simulink model "Q_Car_RL_TD3_Road_Signal"  (R2020b)
settings: Solver=VariableStepAuto  StartTime=0.0  StopTime=4  RelTol=1e-3
values from neighbouring files (symbols this model uses):
  b1 = 2126    [ModelParameters.mat]
  b2 = 1000    [ModelParameters.mat]
  Gqn0 = 4096 X 10^-6 (0.004096)    [RoadParameters.m]
  k1 = 24000    [ModelParameters.mat]
  k2 = 350000    [ModelParameters.mat]
  m1 = 365    [ModelParameters.mat]
  m2 = 43    [ModelParameters.mat]
  P_Noise = 28.5    [RoadParameters.m]
  Ts = 0.001    [Agent_Run.m]    (also in Learning_Algorithm_TD3.m)
undefined symbols (not defined in the file or in its folder): DiscIntNeverNeededParam, magnitude
libraries: simulink x4, rllib x1
settings Model: Creator=Administrator  LastModifiedBy=cloud
settings SolverCC: ZeroCrossAlgorithm=Adaptive
settings DebuggingCC: MaskedZcDiagnostic=none  IgnoredZcDiagnostic=none

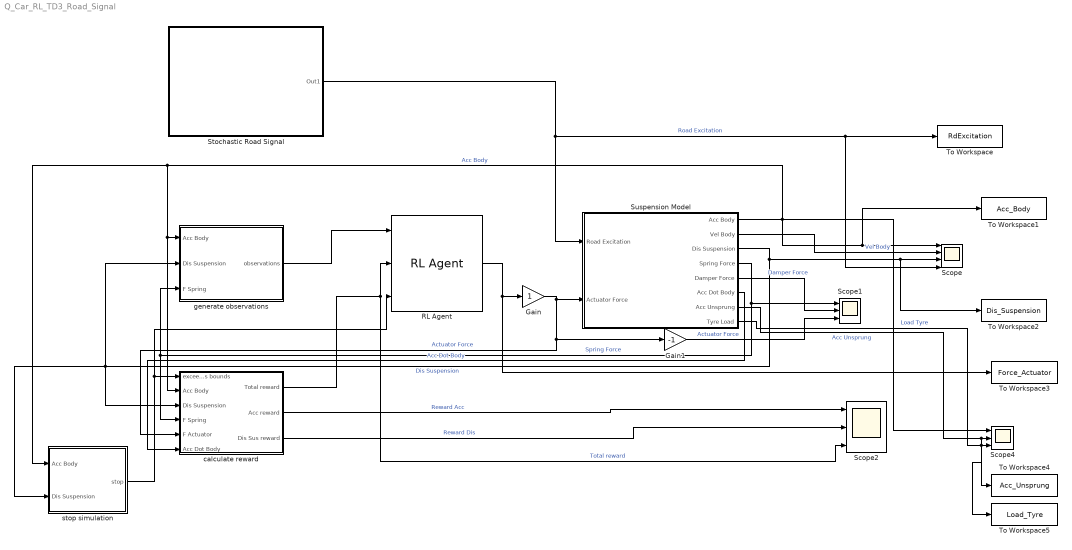
== system Q_Car_RL_TD3_Road_Signal ==
  Gain : Gain
  Gain1 : Gain  Gain=-1
  RL Agent : rllib/RL Agent  Agent=agent  ProvideReward=on  ProvideIsDone=on  ProvideCumRwd=off  TreatAsDirectFeedthrough=on  CollectLoggedSignals=on  CollectModelStates=on
  Scope : Scope  NumInputPorts=4
  Scope1 : Scope  NumInputPorts=3
  Scope2 : Scope  NumInputPorts=3
  Scope4 : Scope  NumInputPorts=3
  Stochastic Road Signal : Subsystem
  Suspension Model : Subsystem
  To Workspace : ToWorkspace  VariableName=RdExcitation  SaveFormat=Timeseries  SampleTime=0.001
  To Workspace1 : ToWorkspace  VariableName=Acc_Body  SaveFormat=Timeseries  SampleTime=0.001
  To Workspace2 : ToWorkspace  VariableName=Dis_Suspension  SaveFormat=Timeseries  SampleTime=0.001
  To Workspace3 : ToWorkspace  VariableName=Force_Actuator  SaveFormat=Structure With Time  SampleTime=0.001
  To Workspace4 : ToWorkspace  VariableName=Acc_Unsprung  SaveFormat=Timeseries  SampleTime=0.001
  To Workspace5 : ToWorkspace  VariableName=Load_Tyre  SaveFormat=Structure With Time  SampleTime=0.001
  calculate reward : Subsystem
  generate observations : Subsystem
  stop simulation : Subsystem
  wires:
  Suspension Model/1(Acc Body) -> Scope/1, To Workspace1/1, calculate reward/2(Acc Body), generate observations/1(Acc Body), stop simulation/1(Acc Body), Scope4/1  "Acc Body"
  Suspension Model/3(Dis Suspension) -> Scope/3, To Workspace2/1, calculate reward/3(Dis Suspension), stop simulation/2(Dis Suspension), generate observations/2(Dis Suspension)  "Dis Suspension"
  Stochastic Road Signal/1(Out1) -> To Workspace/1, Scope/4, Suspension Model/1(Road Excitation)  "Road Excitation"
  generate observations/1(observations) -> RL Agent/1
  calculate reward/1(Total reward) -> Scope2/3, RL Agent/2  "Total reward"
  stop simulation/1(stop) -> calculate reward/1(exceeds bounds), RL Agent/3
  RL Agent/1 -> Gain/1, To Workspace3/1
  Gain/1 -> Gain1/1, calculate reward/5(F Actuator), Suspension Model/2(Actuator Force)  "Actuator Force"
  Suspension Model/4(Spring Force) -> calculate reward/4(F Spring), generate observations/3(F Spring), Scope1/1  "Spring Force"
  Suspension Model/5(Damper Force) -> Scope1/2  "Damper Force"
  Suspension Model/6(Acc Dot Body) -> calculate reward/6(Acc Dot Body)  "Acc Dot Body"
  calculate reward/2(Acc reward) -> Scope2/1  "Reward Acc"
  calculate reward/3(Dis Sus reward) -> Scope2/2  "Reward Dis"
  Gain1/1 -> Scope1/3  "Actuator Force"
  Suspension Model/2(Vel Body) -> Scope/2  "Vel Body"
  Suspension Model/7(Acc Unsprung) -> To Workspace4/1, Scope4/2  "Acc Unsprung"
  Suspension Model/8(Tyre Load) -> To Workspace5/1, Scope4/3  "Load Tyre"

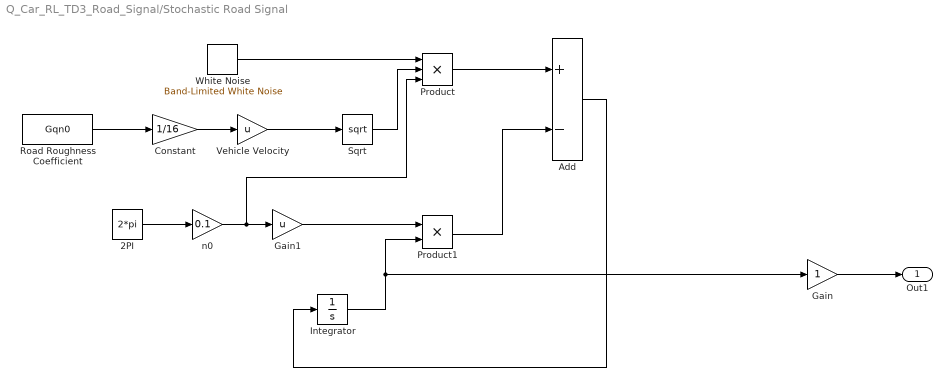
== system Q_Car_RL_TD3_Road_Signal/Stochastic Road Signal ==
  2PI : Constant  Value=2*pi
  Add : Sum  Inputs=+-
  Constant : Gain  Gain=1/16
  Gain : Gain
  Gain1 : Gain  Gain=u
  Integrator : Integrator
  Product : Product  Inputs=3
  Product1 : Product
  Road Roughness Coefficient : Constant  Value=Gqn0
  Sqrt : Sqrt  SaturateOnIntegerOverflow=on
  Vehicle Velocity : Gain  Gain=u
  White Noise : simulink/Sources/Band-Limited White Noise  Cov=[P_Noise]  Ts=0.001  seed=[23341]
  n0 : Gain  Gain=0.1
  Out1 : Outport
  wires:
  Integrator/1 -> Product1/2, Gain/1
  White Noise/1 -> Product/1
  2PI/1 -> n0/1
  n0/1 -> Product/3, Gain1/1
  Gain1/1 -> Product1/1
  Road Roughness Coefficient/1 -> Constant/1
  Gain/1 -> Out1/1
  Constant/1 -> Vehicle Velocity/1
  Add/1 -> Integrator/1
  Product/1 -> Add/1
  Product1/1 -> Add/2
  Sqrt/1 -> Product/2
  Vehicle Velocity/1 -> Sqrt/1

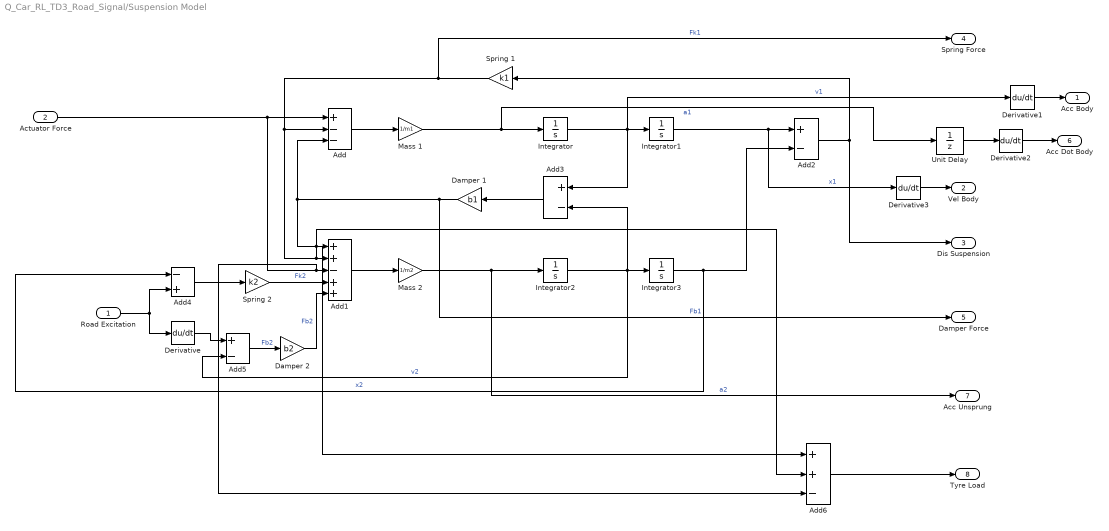
== system Q_Car_RL_TD3_Road_Signal/Suspension Model ==
  Road Excitation : Inport
  Actuator Force : Inport  Port=2
  Add : Sum  Inputs=+--
  Add1 : Sum  Inputs=++-++
  Add2 : Sum  Inputs=+-
  Add3 : Sum  Inputs=+-
  Add4 : Sum  Inputs=-+
  Add5 : Sum  Inputs=+-
  Add6 : Sum  Inputs=++-
  Damper 1 : Gain  Gain=b1
  Damper 2 : Gain  Gain=b2
  Derivative{,1..3} (4 alike) : Derivative
  Integrator{,1..3} (4 alike) : Integrator
  Mass 1 : Gain  Gain=1/m1
  Mass 2 : Gain  Gain=1/m2
  Spring 1 : Gain  Gain=k1
  Spring 2 : Gain  Gain=k2
  Unit Delay : UnitDelay  SampleTime=-1  HasFrameUpgradeWarning=on
  Acc Body : Outport
  Vel Body : Outport  Port=2
  Dis Suspension : Outport  Port=3
  Spring Force : Outport  Port=4
  Damper Force : Outport  Port=5
  Acc Dot Body : Outport  Port=6
  Acc Unsprung : Outport  Port=7
  Tyre Load : Outport  Port=8
  wires:
  Road Excitation/1 -> Derivative/1, Add4/2
  Actuator Force/1 -> Add/1, Add6/3, Add1/3
  Add/1 -> Mass 1/1
  Add5/1 -> Damper 2/1  "Fb2"
  Damper 2/1 -> Add1/5  "Fb2"
  Integrator/1 -> Derivative1/1, Add3/1, Integrator1/1  "v1"
  Add3/1 -> Damper 1/1
  Damper 1/1 -> Damper Force/1, Add6/1, Add1/1, Add/3  "Fb1"
  Add1/1 -> Mass 2/1
  Integrator1/1 -> Derivative3/1, Add2/1  "x1"
  Add4/1 -> Spring 2/1
  Integrator3/1 -> Add4/1, Add2/2  "x2"
  Spring 2/1 -> Add1/4  "Fk2"
  Spring 1/1 -> Spring Force/1, Add/2, Add6/2, Add1/2  "Fk1"
  Mass 1/1 -> Unit Delay/1, Integrator/1  "a1"
  Integrator2/1 -> Add5/2, Add3/2, Integrator3/1  "v2"
  Mass 2/1 -> Integrator2/1, Acc Unsprung/1  "a2"
  Derivative/1 -> Add5/1
  Add2/1 -> Dis Suspension/1, Spring 1/1
  Derivative3/1 -> Vel Body/1
  Derivative1/1 -> Acc Body/1
  Derivative2/1 -> Acc Dot Body/1
  Unit Delay/1 -> Derivative2/1
  Add6/1 -> Tyre Load/1

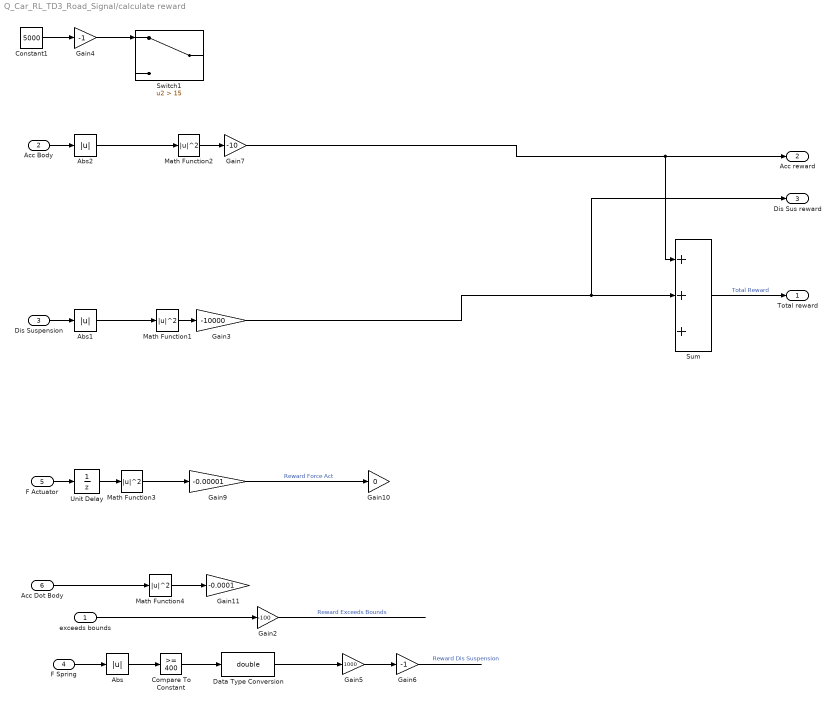
== system Q_Car_RL_TD3_Road_Signal/calculate reward ==
  exceeds bounds : Inport
  Acc Body : Inport  Port=2
  Dis Suspension : Inport  Port=3
  F Spring : Inport  Port=4
  F Actuator : Inport  Port=5
  Acc Dot Body : Inport  Port=6
  Abs : Abs
  Abs1 : Abs
  Abs2 : Abs
  Compare To Constant : simulink/Logic and Bit Operations/Compare To Constant  relop=>=  const=400  OutDataTypeStr=boolean
  Constant1 : Constant  Value=5000
  Data Type Conversion : DataTypeConversion  OutDataTypeStr=double
  Gain10 : Gain  Gain=0
  Gain11 : Gain  Gain=-0.0001
  Gain2 : Gain  Gain=-100
  Gain3 : Gain  Gain=-10000
  Gain4 : Gain  Gain=-1
  Gain5 : Gain  Gain=1000
  Gain6 : Gain  Gain=-1
  Gain7 : Gain  Gain=-10
  Gain9 : Gain  Gain=-0.00001
  Math Function{1..4} (4 alike) : Math  Operator=magnitude^2  SaturateOnIntegerOverflow=on
  Sum : Sum  Inputs=+++  OutDataTypeStr=double
  Switch1 : Switch  Criteria=u2 > Threshold  Threshold=15
  Unit Delay : UnitDelay  SampleTime=Ts  HasFrameUpgradeWarning=on
  Total reward : Outport  VectorParamsAs1DForOutWhenUnconnected=off
  Acc reward : Outport  Port=2  VectorParamsAs1DForOutWhenUnconnected=off
  Dis Sus reward : Outport  Port=3  VectorParamsAs1DForOutWhenUnconnected=off
  wires:
  Gain2/1 -> ?  "Reward Exceeds Bounds"
  exceeds bounds/1 -> Gain2/1
  F Spring/1 -> Abs/1
  Gain5/1 -> Gain6/1
  Gain6/1 -> ?  "Reward Dis Suspension"
  Compare To Constant/1 -> Data Type Conversion/1
  Data Type Conversion/1 -> Gain5/1
  Abs/1 -> Compare To Constant/1
  Sum/1 -> Total reward/1  "Total Reward"
  Math Function1/1 -> Gain3/1
  Abs1/1 -> Math Function1/1
  Dis Suspension/1 -> Abs1/1
  Math Function2/1 -> Gain7/1
  Acc Body/1 -> Abs2/1
  Abs2/1 -> Math Function2/1
  Constant1/1 -> Gain4/1
  Unit Delay/1 -> Math Function3/1
  Math Function3/1 -> Gain9/1
  F Actuator/1 -> Unit Delay/1
  Gain9/1 -> Gain10/1  "Reward Force Act"
  Acc Dot Body/1 -> Math Function4/1
  Math Function4/1 -> Gain11/1
  Gain3/1 -> Sum/2, Dis Sus reward/1
  Gain4/1 -> Switch1/1
  Gain7/1 -> Sum/1, Acc reward/1

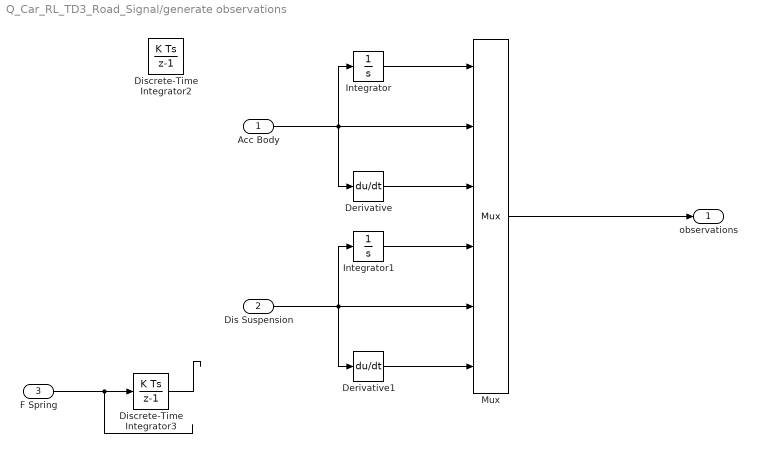
== system Q_Car_RL_TD3_Road_Signal/generate observations ==
  Acc Body : Inport
  Dis Suspension : Inport  Port=2
  F Spring : Inport  Port=3
  Derivative : Derivative
  Derivative1 : Derivative
  Discrete-Time Integrator2 : DiscreteIntegrator  SampleTime=Ts  ICPrevOutput=DiscIntNeverNeededParam  ICPrevScaledInput=DiscIntNeverNeededParam
  Discrete-Time Integrator3 : DiscreteIntegrator  SampleTime=Ts  ICPrevOutput=DiscIntNeverNeededParam  ICPrevScaledInput=DiscIntNeverNeededParam
  Integrator : Integrator
  Integrator1 : Integrator
  Mux : Mux  Inputs=6
  observations : Outport  VectorParamsAs1DForOutWhenUnconnected=off
  wires:
  Mux/1 -> observations/1
  Acc Body/1 -> Integrator/1, Mux/2, Derivative/1
  Discrete-Time Integrator3/1 -> ?
  F Spring/1 -> Discrete-Time Integrator3/1
  Dis Suspension/1 -> Integrator1/1, Mux/5, Derivative1/1
  Integrator/1 -> Mux/1
  Derivative/1 -> Mux/3
  Integrator1/1 -> Mux/4
  Derivative1/1 -> Mux/6

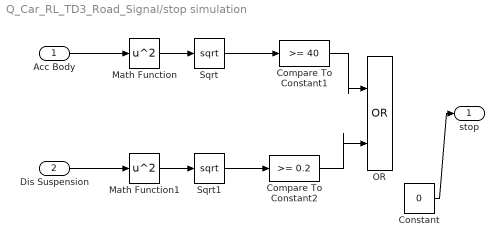
== system Q_Car_RL_TD3_Road_Signal/stop simulation ==
  Acc Body : Inport
  Dis Suspension : Inport  Port=2
  Compare To Constant1 : simulink/Logic and Bit Operations/Compare To Constant  relop=>=  const=40  OutDataTypeStr=boolean
  Compare To Constant2 : simulink/Logic and Bit Operations/Compare To Constant  relop=>=  const=0.2  OutDataTypeStr=boolean
  Constant : Constant  Value=0
  Math Function : Math  Operator=square  SaturateOnIntegerOverflow=on
  Math Function1 : Math  Operator=square  SaturateOnIntegerOverflow=on
  OR : Logic  Operator=OR  IconShape=distinctive  AllPortsSameDT=off  OutDataTypeStr=boolean
  Sqrt : Sqrt  SaturateOnIntegerOverflow=on
  Sqrt1 : Sqrt  SaturateOnIntegerOverflow=on
  stop : Outport  VectorParamsAs1DForOutWhenUnconnected=off
  wires:
  Compare To Constant1/1 -> OR/1
  Compare To Constant2/1 -> OR/2
  Math Function/1 -> Sqrt/1
  Math Function1/1 -> Sqrt1/1
  Sqrt/1 -> Compare To Constant1/1
  Acc Body/1 -> Math Function/1
  Dis Suspension/1 -> Math Function1/1
  Sqrt1/1 -> Compare To Constant2/1
  Constant/1 -> stop/1
